simulink model "EKF_SIL_02_newdelIpsOOSM"  (R2014a)
settings: Solver=ode45  StartTime=0.0  StopTime=50  RelTol=1e-3
model workspace: external: MATLAB File InitOOSM.m (data not in the file)
undefined symbols (not defined in the file): Cov_nu, Cov_r, e_force_x, e_force_y, e_force_z, ieps, ita, n, P_0, P_k, p_x, p_y, p_z, parameter_gravitation, rho, rho_c, sig_f, sig_tau, t_delta, t_Kalman, t_RobotSense, tau_1, tau_2, tau_3, U_n_d, X_a_0, x_k
libraries: simulink x9, dspmtrx3 x4, aerolibtransform2 x2, visionsinks x1
(part 3 of 6)

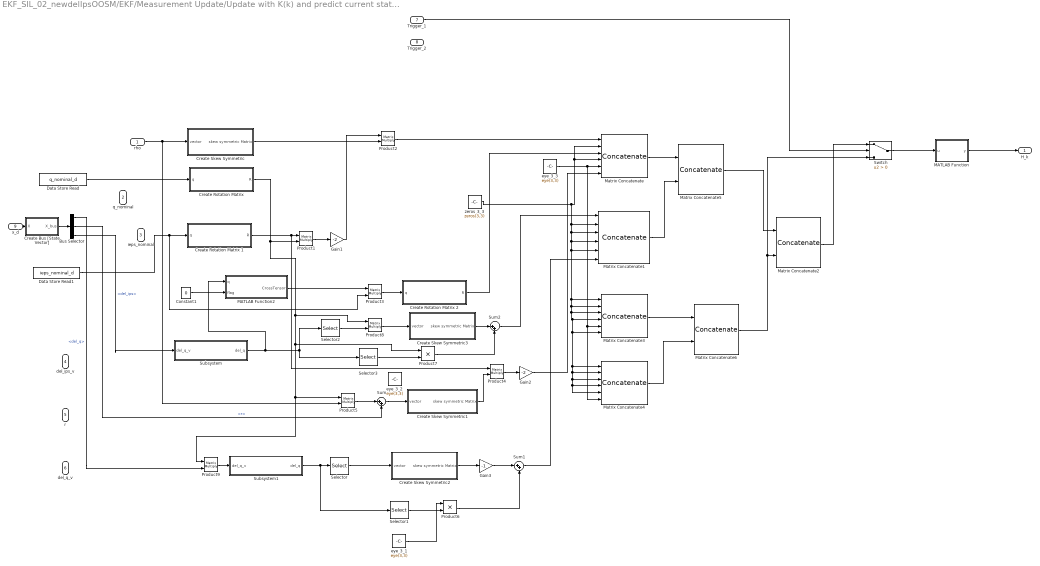
== system EKF_SIL_02_newdelIpsOOSM/EKF/Measurement Update/Update with K(k) and predict current state/Create H_k ==
  rho : Inport
  q_nominal : Inport  Port=2
  ieps_nominal : Inport  Port=3
  del_ips_v : Inport  Port=4
  r : Inport  Port=5
  del_q_v : Inport  Port=6
  Trigger_1 : Inport  Port=7
  Trigger_2 : Inport  Port=8
  x_d : Inport  Port=9
  Bus Selector : BusSelector  OutputSignals=del_q,r,del_ips
  Constant1 : Constant  Value=0
  Create Bus [State Vector] : Subsystem
  "Create Rotation Matrix " : Subsystem
  Create Rotation Matrix 1 : Subsystem
  Create Rotation Matrix 2 : Subsystem
  Create Skew Symmetric : Subsystem
  Create Skew Symmetric1 : Subsystem
  Create Skew Symmetric2 : Subsystem
  Create Skew Symmetric3 : Subsystem
  Data Store Read : DataStoreRead  DataStoreName=q_nominal_d
  Data Store Read1 : DataStoreRead  DataStoreName=ieps_nominal_d
  Gain1 : Gain  Gain=-2
  Gain2 : Gain  Gain=-2
  Gain3 : Gain  Gain=-1
  MATLAB Function : MATLAB Function  TreatAsAtomicUnit=on
      settings: PermitHierarchicalResolution=ParametersOnly
  MATLAB Function2 : MATLAB Function  TreatAsAtomicUnit=on
      settings: PermitHierarchicalResolution=ParametersOnly
  Matrix Concatenate{,1,3..4} (4 alike) : Concatenate  NumInputs=6  Mode=Multidimensional array  ConcatenateDimension=2
  Matrix Concatenate2 : Concatenate  Mode=Multidimensional array
  Matrix Concatenate5 : Concatenate  Mode=Multidimensional array
  Matrix Concatenate6 : Concatenate  Mode=Multidimensional array
  Product{1..5,8..9} (7 alike) : Product  Multiplication=Matrix(*)
  Product6 : Product
  Product7 : Product
  Selector : Selector  InputPortWidth=4  Indices=[1:3]
  Selector1 : Selector  InputPortWidth=4  Indices=4
  Selector2 : Selector  InputPortWidth=4  Indices=[1:3]
  Selector3 : Selector  InputPortWidth=4  Indices=4
  Subsystem : Subsystem
  Subsystem1 : Subsystem
  Sum : Sum  Inputs=|++
  Sum1 : Sum  Inputs=|++
  Sum2 : Sum  Inputs=|++
  Switch : Switch  Criteria=u2 > Threshold  AllowDiffInputSizes=on
  eye_3_1 : Constant  Value=eye(3,3)
  eye_3_2 : Constant  Value=eye(3,3)
  eye_3_3 : Constant  Value=eye(3,3)
  zeros_3_3 : Constant  Value=zeros(3,3)
  H_k : Outport
  wires:
  Data Store Read/1 -> "Create Rotation Matrix "/1(q)
  Switch/1 -> MATLAB Function/1(u)
  eye_3_3/1 -> Matrix Concatenate4/6, Matrix Concatenate3/5, Matrix Concatenate/5
  Create Skew Symmetric/1(skew symmetric Matrix) -> Product2/2
  rho/1 -> Product5/2, Create Skew Symmetric/1(vector)
  Create Rotation Matrix 1/1(R) -> Product4/1, Product1/1
  Product1/1 -> Gain1/1
  Gain1/1 -> Product2/1
  Product2/1 -> Matrix Concatenate/1
  Bus Selector/3 -> Subsystem/1(del_q_v)  "<del_ips>"
  Constant1/1 -> MATLAB Function2/2(flag)
  MATLAB Function2/1(CrossTensor) -> Product3/1
  Data Store Read1/1 -> Product3/2, Create Rotation Matrix 1/1(q)
  Create Rotation Matrix 2/1(R) -> Matrix Concatenate/3
  "Create Rotation Matrix "/1(R) -> Product7/1, Product9/1, Product5/1, Product8/1, Product1/2
  Product5/1 -> Sum/1
  Bus Selector/2 -> Sum/2  "<r>"
  Gain2/1 -> Matrix Concatenate/6
  Subsystem1/1(del_q) -> Selector1/1, Selector/1
  Selector/1 -> Create Skew Symmetric2/1(vector)
  Create Skew Symmetric2/1(skew symmetric Matrix) -> Gain3/1
  Selector1/1 -> Product6/2
  eye_3_1/1 -> Product6/1
  Gain3/1 -> Sum1/1
  Product6/1 -> Sum1/2
  Sum1/1 -> Matrix Concatenate1/6
  Selector2/1 -> Product8/2
  Create Skew Symmetric3/1(skew symmetric Matrix) -> Sum2/1
  Selector3/1 -> Product7/2
  Product7/1 -> Sum2/2
  Sum2/1 -> Matrix Concatenate1/1
  Sum/1 -> Create Skew Symmetric1/1(vector)
  Create Skew Symmetric1/1(skew symmetric Matrix) -> Product4/2
  Product3/1 -> Create Rotation Matrix 2/1(q)
  zeros_3_3/1 -> Matrix Concatenate3/6, Matrix Concatenate4/1, Matrix Concatenate4/5, Matrix Concatenate4/4, Matrix Concatenate4/3, Matrix Concatenate4/2, Matrix Concatenate3/4, Matrix Concatenate3/3, Matrix Concatenate3/2, Matrix Concatenate3/1, Matrix Concatenate1/5, Matrix Concatenate1/4, Matrix Concatenate1/3, Matrix Concatenate1/2, Matrix Concatenate/4, Matrix Concatenate/2
  Matrix Concatenate1/1 -> Matrix Concatenate5/2
  Matrix Concatenate4/1 -> Matrix Concatenate6/2
  Subsystem/1(del_q) -> MATLAB Function2/1(q), Selector2/1, Selector3/1
  Bus Selector/1 -> Product9/2  "<del_q>"
  Product9/1 -> Subsystem1/1(del_q_v)
  Product8/1 -> Create Skew Symmetric3/1(vector)
  Product4/1 -> Gain2/1
  Matrix Concatenate/1 -> Matrix Concatenate5/1
  Matrix Concatenate3/1 -> Matrix Concatenate6/1
  Trigger_1/1 -> Switch/2
  Matrix Concatenate5/1 -> Matrix Concatenate2/1
  Matrix Concatenate6/1 -> Switch/3, Matrix Concatenate2/2
  Matrix Concatenate2/1 -> Switch/1
  MATLAB Function/1(y) -> H_k/1
  Create Bus [State Vector]/1(X_bus) -> Bus Selector/1
  x_d/1 -> Create Bus [State Vector]/1(X)

== system EKF_SIL_02_newdelIpsOOSM/EKF/Measurement Update/Update with K(k) and predict current state/Create S_k ==
  ita_nominal : Inport
  trig_1 : Inport  Port=2
  trig_2 : Inport  Port=3
  q_nominal : Inport  Port=4
  cov_r : Inport  Port=5
  cov_nu : Inport  Port=6
  Constant : Constant  Value=1e-4*eye(6,6)
  Constant1 : Constant  Value=zeros(6,6)
  Data Store Read : DataStoreRead  DataStoreName=q_nominal_d
  Matrix Concatenate1 : Concatenate  Mode=Multidimensional array
  Matrix Concatenate5 : Concatenate  Mode=Multidimensional array  ConcatenateDimension=2
  Matrix Concatenate6 : Concatenate  Mode=Multidimensional array  ConcatenateDimension=2
  Measurement noise covariance : MATLAB Function  TreatAsAtomicUnit=on
      settings: PermitHierarchicalResolution=ParametersOnly
  Switch : Switch  Criteria=u2 > Threshold  AllowDiffInputSizes=on
  S_k : Outport
  wires:
  ita_nominal/1 -> Measurement noise covariance/2(ita_nominal)
  cov_nu/1 -> Measurement noise covariance/4(cov_nu)
  cov_r/1 -> Measurement noise covariance/3(cov_r)
  Measurement noise covariance/1(S) -> Matrix Concatenate5/1, Switch/3
  trig_1/1 -> Switch/2
  Constant1/1 -> Matrix Concatenate6/1, Matrix Concatenate5/2
  Constant/1 -> Matrix Concatenate6/2
  Switch/1 -> S_k/1
  Matrix Concatenate1/1 -> Switch/1
  Matrix Concatenate5/1 -> Matrix Concatenate1/1
  Matrix Concatenate6/1 -> Matrix Concatenate1/2
  Data Store Read/1 -> Measurement noise covariance/1(q_nominal)

== system EKF_SIL_02_newdelIpsOOSM/EKF/Measurement Update/Update with K(k) and predict current state/Create X_a from X ==
  q_nominal : Inport
  X : Inport  Port=2
  ieps_nominal : Inport  Port=3
  Bus Creator1 : BusCreator
  Bus Creator2 : BusCreator  Inputs=6
  Bus Creator3 : BusCreator
  Bus Selector2 : BusSelector  OutputSignals=del_q,del_ips
  Bus Selector3 : BusSelector  OutputSignals=omega,r,r_dot,rho_c
  Create Bus [State Vector] : Subsystem
  "Create q_nominal " : Subsystem
  Create q_nominal 1 : Subsystem
  Demux : Demux
  Demux1 : Demux
  Display2 : Display
  Signal Conversion : SignalConversion
  X_a(k+1) : Outport
  X_a(internal) : Outport  Port=2
  "X(reduced) " : Outport  Port=3
  wires:
  Bus Selector3/3 -> Bus Creator2/4  "<r_dot>"
  Demux/1 -> Bus Creator3/1  "q_est_1"
  Bus Selector3/2 -> Bus Creator2/3  "<r>"
  Bus Creator3/1 -> Bus Creator2/1  "q_est"
  Create Bus [State Vector]/1(X_bus) -> "X(reduced) "/1, Bus Selector3/1, Bus Selector2/1
  X/1 -> Create Bus [State Vector]/1(X)
  Bus Selector3/1 -> Bus Creator2/2  "<omega>"
  Demux/2 -> Bus Creator3/2  "q_est_2"
  Demux/4 -> Bus Creator3/4  "q_est_0"
  Demux/3 -> Bus Creator3/3  "q_est_3"
  Bus Selector2/1 -> "Create q_nominal "/1(del_q)  "<del_q>"
  q_nominal/1 -> "Create q_nominal "/2(q_nominal)
  "Create q_nominal "/1(q_est) -> Demux/1
  Bus Creator2/1 -> Signal Conversion/1, X_a(internal)/1
  Bus Selector2/2 -> Create q_nominal 1/1(del_q)  "<del_ips>"
  ieps_nominal/1 -> Create q_nominal 1/2(q_nominal)
  Bus Selector3/4 -> Bus Creator2/5  "<rho_c>"
  Demux1/1 -> Bus Creator1/1  "ieps_est_1"
  Bus Creator1/1 -> Bus Creator2/6  "ieps_est"
  Demux1/2 -> Bus Creator1/2  "ieps_est_2"
  Demux1/4 -> Bus Creator1/4  "ieps_est_0"
  Demux1/3 -> Bus Creator1/3  "ieps_est_3"
  Create q_nominal 1/1(q_est) -> Display2/1, Demux1/1
  Signal Conversion/1 -> X_a(k+1)/1

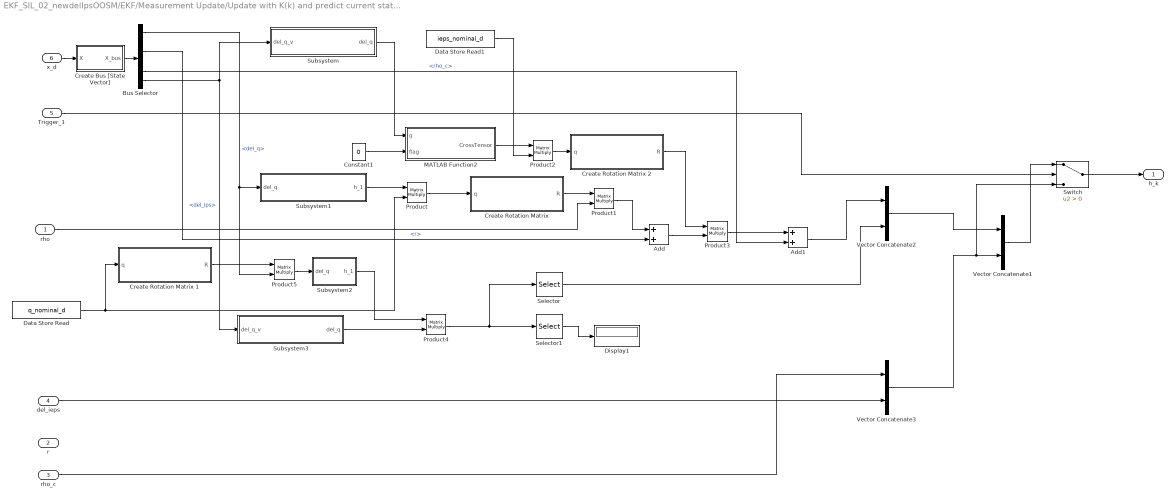
== system EKF_SIL_02_newdelIpsOOSM/EKF/Measurement Update/Update with K(k) and predict current state/Create h ==
  rho : Inport
  r : Inport  Port=2
  rho_c : Inport  Port=3
  "del_ieps " : Inport  Port=4
  Trigger_1 : Inport  Port=5
  x_d : Inport  Port=6
  Add : Sum
  Add1 : Sum
  Bus Selector : BusSelector  OutputSignals=del_q,omega,r,r_dot,rho_c,del_ips
  Constant1 : Constant  Value=0
  Create Bus [State Vector] : Subsystem
  "Create Rotation Matrix " : Subsystem
  Create Rotation Matrix 1 : Subsystem
  Create Rotation Matrix 2 : Subsystem
  Data Store Read : DataStoreRead  DataStoreName=q_nominal_d
  Data Store Read1 : DataStoreRead  DataStoreName=ieps_nominal_d
  Display1 : Display
  MATLAB Function2 : MATLAB Function  TreatAsAtomicUnit=on
      settings: PermitHierarchicalResolution=ParametersOnly
  Product{,1..5} (6 alike) : Product  Multiplication=Matrix(*)
  Selector : Selector  InputPortWidth=4  Indices=[1:3]
  Selector1 : Selector  InputPortWidth=4  Indices=4
  Subsystem : Subsystem
  Subsystem1 : Subsystem
  Subsystem2 : Subsystem
  Subsystem3 : Subsystem
  Switch : Switch  Criteria=u2 > Threshold  AllowDiffInputSizes=on
  Vector Concatenate1 : Concatenate
  Vector Concatenate2 : Concatenate
  Vector Concatenate3 : Concatenate
  h_k : Outport
  wires:
  rho/1 -> Product1/2
  Data Store Read/1 -> Product/2, Create Rotation Matrix 1/1(q)
  "Create Rotation Matrix "/1(R) -> Product1/1
  Product/1 -> "Create Rotation Matrix "/1(q)
  Subsystem1/1(h_1) -> Product/1
  Product1/1 -> Add/1
  rho_c/1 -> Vector Concatenate3/1
  "del_ieps "/1 -> Vector Concatenate3/2
  Create Rotation Matrix 2/1(R) -> Product3/1
  Product3/1 -> Add1/1
  Add/1 -> Product3/2
  Add1/1 -> Vector Concatenate2/1
  Product4/1 -> Selector1/1, Selector/1
  Selector1/1 -> Display1/1
  Create Rotation Matrix 1/1(R) -> Product5/1
  Product5/1 -> Subsystem2/1(del_q)
  Subsystem2/1(h_1) -> Product4/1
  Selector/1 -> Vector Concatenate2/2
  Trigger_1/1 -> Switch/2
  Vector Concatenate2/1 -> Vector Concatenate1/1
  Vector Concatenate3/1 -> Switch/3, Vector Concatenate1/2
  Switch/1 -> h_k/1
  Vector Concatenate1/1 -> Switch/1
  x_d/1 -> Create Bus [State Vector]/1(X)
  Bus Selector/1 -> Product5/2, Subsystem1/1(del_q)  "<del_q>"
  Bus Selector/3 -> Add/2  "<r>"
  Bus Selector/5 -> Add1/2  "<rho_c>"
  Bus Selector/6 -> Subsystem3/1(del_q_v), Subsystem/1(del_q_v)  "<del_ips>"
  Subsystem3/1(del_q) -> Product4/2
  Create Bus [State Vector]/1(X_bus) -> Bus Selector/1
  Constant1/1 -> MATLAB Function2/2(flag)
  Subsystem/1(del_q) -> MATLAB Function2/1(q)
  MATLAB Function2/1(CrossTensor) -> Product2/1
  Product2/1 -> Create Rotation Matrix 2/1(q)
  Data Store Read1/1 -> Product2/2

== matlab function EKF_SIL_02_newdelIpsOOSM/EKF/OOSM_KF/OOSM_KF/State Propagation/MATLAB Function ==
  data: X_a input; Phi output; n input; t_Kalman input; p input; M input; V input; om_EE input
%Function: fn_Create_Phi()
%Inputs: X_a - 23-state vector,
%        n - angular velocity of spacecrafts,
%        t_delta - sampling time
%Outputs: [Phi] (State-propagation Matrix)
%Functionality: Generates the State Propagation matrix
%Author: Hrishik Mishra
function Phi  = fn_Create_Phi(X_a,n,t_Kalman,p,M,V,om_EE)
    Phi_t = fn_Create_Phi_t(n,t_Kalman);
    Phi_r = fn_Create_Phi_r(X_a,p, t_Kalman);    
    Phi_rho_c = expm(fn_VectorToSkewSymmetricTensor(V(4:6))*t_Kalman);
    Phi_ieps = expm(-fn_VectorToSkewSymmetricTensor(om_EE*t_Kalman));
    Phi_robot = [Phi_rho_c,zeros(3,3);zeros(3,3),Phi_ieps];
    
    Phi = [Phi_r, zeros(6,12);zeros(6,6),Phi_t,zeros(6,6);zeros(6,12),Phi_robot];

end
%Create state propagation matrix of the whole system

%Function: fn_Create_Phi_r()
%Inputs: X_a - 23-state vector,
%Outputs: [Phi_r] (State-propagation Matrix for Rotation component)
%Functionality: Generates the State Propagation matrix for Rotation
%component
%Author: Hrishik Mishra
function [Phi_r] = fn_Create_Phi_r(X_a,p,t_Kalman) 
    Phi_r = zeros(6,6);
    omega = X_a(5:7);
    M = fn_Create_M(p,omega);   
    
    A = [-fn_VectorToSkewSymmetricTensor(omega),0.5*eye(3,3);zeros(3,3),M];
    Phi_r = expm(A*t_Kalman);
%     phi_r11 = fn_Create_phi_r11(omega,t_delta);
%     phi_r12 = fn_Create_phi_r12(omega,M,t_delta);
%     phi_r22 = fn_Create_phi_r22(omega,t_delta,M);
%     phi_r13 = fn_Create_phi_r13(omega,t_delta,M,N);
%     phi_r23 = fn_Create_phi_r23(omega,t_delta,M,N);
%     Phi_r = [phi_r11, phi_r12, phi_r13;zeros(3,3),phi_r22,phi_r23;zeros(3,3),zeros(3,3),eye(3,3)];
%     

end
%Function: fn_Create_M()
%Inputs: p - Inertial ratios 
%        omega - angular velocity between Chaser Grasping frame and Chaser
%        CoM
%Outputs: M (Linearized model matrix for inertial parameters)
%Functionality: Generates M
%Author: Hrishik Mishra
function M = fn_Create_M(p,omega)
    %#Codegen
    
    M = [0, p(1)*omega(3), p(1)*omega(2); p(2)*omega(3), 0, p(2)*omega(1); p(3)*omega(2),p(3)*omega(1),0];
end
%Function: fn_Create_N()
%Inputs: omega - angular velocity between Chaser Grasping frame and Chaser
%        CoM
%Outputs: N (Linearized model matrix for inertial parameters)
%Functionality: Generates M
%Author: Hrishik Mishra
function N = fn_Create_N(omega)
%
    N = [omega(2)*omega(3), 0, 0; 0, omega(1)*omega(3), 0; 0, 0, omega(1)*omega(2)];
end

%%
%Function: fn_Create_Phi_t()
%Inputs: n - angular velocity of Chaser/Target (almost same)
%        t_delta - sampling time
%Outputs: Phi_t (State Transition Matrix for Translation component)
%Functionality: Generates Phi_t
%Author: Hrishik Mishra
function Phi_t = fn_Create_Phi_t(n,t_delta)
%
    Phi_t12 = [t_delta, n*t_delta^2,0;0, t_delta, 0;0,0,t_delta];
    Phi_t22 = eye(3,3) - 2*fn_VectorToSkewSymmetricTensor([0;0;n])*t_delta;
    
    Phi_t = [eye(3,3),Phi_t12;zeros(3,3),Phi_t22];
    
end

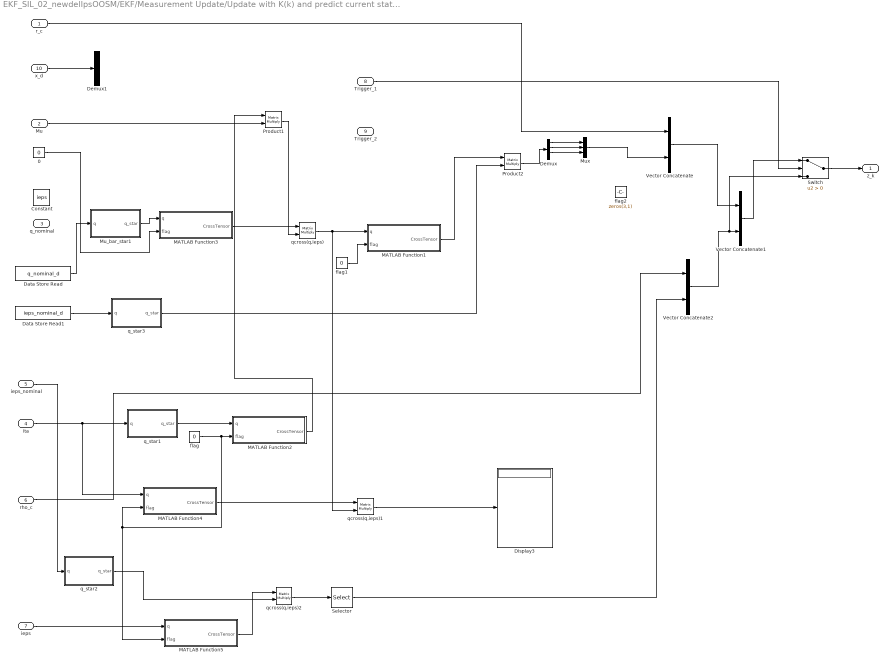
== system EKF_SIL_02_newdelIpsOOSM/EKF/Measurement Update/Update with K(k) and predict current state/Create observation ==
  r_c : Inport
  Mu : Inport  Port=2
  q_nominal : Inport  Port=3
  ita : Inport  Port=4
  ieps_nominal : Inport  Port=5
  rho_c : Inport  Port=6
  ieps : Inport  Port=7
  Trigger_1 : Inport  Port=8
  Trigger_2 : Inport  Port=9
  x_d : Inport  Port=10
  0 : Constant  Value=0
  Constant : Constant  Value=ieps
  Data Store Read : DataStoreRead  DataStoreName=q_nominal_d
  Data Store Read1 : DataStoreRead  DataStoreName=ieps_nominal_d
  Demux : Demux
  Demux1 : Demux  Outputs=6
  Display3 : Display
  MATLAB Function1 : MATLAB Function  TreatAsAtomicUnit=on
      settings: PermitHierarchicalResolution=ParametersOnly
  MATLAB Function2 : MATLAB Function  TreatAsAtomicUnit=on
      settings: PermitHierarchicalResolution=ParametersOnly
  MATLAB Function3 : MATLAB Function  TreatAsAtomicUnit=on
      settings: PermitHierarchicalResolution=ParametersOnly
  MATLAB Function4 : MATLAB Function  TreatAsAtomicUnit=on
      settings: PermitHierarchicalResolution=ParametersOnly
  MATLAB Function5 : MATLAB Function  TreatAsAtomicUnit=on
      settings: PermitHierarchicalResolution=ParametersOnly
  Mu_bar_star1 : Subsystem
  Mux : Mux  Inputs=3
  Product1 : Product  Multiplication=Matrix(*)
  Product2 : Product  Multiplication=Matrix(*)
  Selector : Selector  InputPortWidth=4  Indices=[1:3]
  Switch : Switch  Criteria=u2 > Threshold  AllowDiffInputSizes=on
  Vector Concatenate : Concatenate
  Vector Concatenate1 : Concatenate
  Vector Concatenate2 : Concatenate
  flag : Constant  Value=0
  flag1 : Constant  Value=0
  flag2 : Constant  Value=zeros(3,1)
  q_star1 : Subsystem
  q_star2 : Subsystem
  q_star3 : Subsystem
  qcross(q,ieps) : Product  Multiplication=Matrix(*)
  qcross(q,ieps)1 : Product  Multiplication=Matrix(*)
  qcross(q,ieps)2 : Product  Multiplication=Matrix(*)
  z_k : Outport
  wires:
  MATLAB Function2/1(CrossTensor) -> Product1/1
  flag/1 -> MATLAB Function2/2(flag), MATLAB Function4/2(flag), MATLAB Function5/2(flag)
  q_star1/1(q_star) -> MATLAB Function2/1(q)
  ita/1 -> MATLAB Function4/1(q), q_star1/1(q)
  Demux/1 -> Mux/1
  Demux/2 -> Mux/2
  Demux/3 -> Mux/3
  Mux/1 -> Vector Concatenate/2
  0/1 -> MATLAB Function3/2(flag)
  r_c/1 -> Vector Concatenate/1
  MATLAB Function1/1(CrossTensor) -> Product2/1
  Product2/1 -> Demux/1
  MATLAB Function3/1(CrossTensor) -> qcross(q,ieps)/1
  ieps_nominal/1 -> q_star2/1(q)
  qcross(q,ieps)/1 -> qcross(q,ieps)1/2, MATLAB Function1/1(q)
  Mu/1 -> Product1/2
  MATLAB Function4/1(CrossTensor) -> qcross(q,ieps)1/1
  qcross(q,ieps)1/1 -> Display3/1
  flag1/1 -> MATLAB Function1/2(flag)
  rho_c/1 -> Vector Concatenate2/1
  q_star2/1(q_star) -> qcross(q,ieps)2/2
  MATLAB Function5/1(CrossTensor) -> qcross(q,ieps)2/1
  ieps/1 -> MATLAB Function5/1(q)
  qcross(q,ieps)2/1 -> Selector/1
  Selector/1 -> Vector Concatenate2/2
  Mu_bar_star1/1(q_star) -> MATLAB Function3/1(q)
  Product1/1 -> qcross(q,ieps)/2
  Vector Concatenate/1 -> Vector Concatenate1/1
  Trigger_1/1 -> Switch/2
  Vector Concatenate2/1 -> Switch/3, Vector Concatenate1/2
  Switch/1 -> z_k/1
  Vector Concatenate1/1 -> Switch/1
  x_d/1 -> Demux1/1
  Data Store Read/1 -> Mu_bar_star1/1(q)
  q_star3/1(q_star) -> Product2/2
  Data Store Read1/1 -> q_star3/1(q)

== system EKF_SIL_02_newdelIpsOOSM/EKF/Measurement Update/Update with K(k) and predict current state/K*H ==
  H : Inport
  K : Inport  Port=2
  Sd : Inport  Port=3
  MATLAB Function : MATLAB Function  TreatAsAtomicUnit=on
      settings: PermitHierarchicalResolution=ParametersOnly
  K*Sd*K' : Outport
  wires:
  K/1 -> MATLAB Function/1(K)
  MATLAB Function/1(y) -> K*Sd*K'/1
  Sd/1 -> MATLAB Function/2(Sd)

== system EKF_SIL_02_newdelIpsOOSM/EKF/Measurement Update/Update with K(k) and predict current state/Kalman gain ==
  H_k : Inport
  P_pre : Inport  Port=2
  S_k : Inport  Port=3
  P_d : Inport  Port=4
  U : Inport  Port=5
  UF : Inport  Port=6
  trig_1 : Inport  Port=7
  Display3 : Display
  MATLAB Function : MATLAB Function  TreatAsAtomicUnit=on
      settings: PermitHierarchicalResolution=ParametersOnly
  Math Function1 : Math  Operator=log10  SaturateOnIntegerOverflow=on
  Scope : Scope
      settings: YMin=-1.61  YMax=-1.41  SaveName=ScopeData22
  Selector : Selector  NumberOfDimensions=2  InputPortWidth=3  IndexOptions=Index vector (dialog),Index vector (dialog)  Indices=[1:6],[1:6]  OutputSizes=1,1
  Sum of Elements : Sum  Inputs=+
  K : Outport
  H.P(k|k-1).H' + S_k : Outport  Port=2
  wires:
  H_k/1 -> MATLAB Function/1(H)
  P_pre/1 -> MATLAB Function/2(P_pre)
  Selector/1 -> Sum of Elements/1
  Sum of Elements/1 -> Math Function1/1
  Math Function1/1 -> Scope/1
  S_k/1 -> MATLAB Function/3(S_k)
  MATLAB Function/1(K) -> K/1
  MATLAB Function/2(Cov_x_y) -> Selector/1, H.P(k|k-1).H' + S_k/1
  P_d/1 -> MATLAB Function/5(P_d)
  U/1 -> MATLAB Function/7(U)
  UF/1 -> MATLAB Function/4(UF)
  trig_1/1 -> MATLAB Function/6(trig_1)

== system EKF_SIL_02_newdelIpsOOSM/EKF/Measurement Update/Update with K(k) and predict current state/MhDist ==
  x : Inport
  Var : Inport  Port=2
  MATLAB Function : MATLAB Function  TreatAsAtomicUnit=on
      settings: PermitHierarchicalResolution=ParametersOnly
  d^2 : Outport
  wires:
  MATLAB Function/1(y) -> d^2/1
  x/1 -> MATLAB Function/1(x)
  Var/1 -> MATLAB Function/2(Var)

== system EKF_SIL_02_newdelIpsOOSM/EKF/Measurement Update/Update with K(k) and predict current state/Outlier rejector ==
  Computed K : Inport
  X^2 : Inport  Port=2
  Chi_threshold : Constant  Value=1000
  Relational Operator : RelationalOperator  Operator=<  OutDataTypeStr=boolean
  Scope : Scope
      settings: ShowLegends=on  SaveName=ScopeData31
  Switch : Switch  Criteria=u2 > Threshold
  zeros(12,) : Constant  Value=zeros(12,6)
  K (outlier_checked) : Outport
  wires:
  Computed K/1 -> Switch/1
  X^2/1 -> Relational Operator/1
  Chi_threshold/1 -> Relational Operator/2
  Relational Operator/1 -> Switch/2, Scope/1  "Outlier rejector (Not)"
  Switch/1 -> K (outlier_checked)/1
  zeros(12,)/1 -> Switch/3

== system EKF_SIL_02_newdelIpsOOSM/EKF/Measurement Update/Update with K(k) and predict current state/Subsystem ==
  residual : Inport
  K : Inport  Port=2
  MATLAB Function : MATLAB Function  TreatAsAtomicUnit=on
      settings: PermitHierarchicalResolution=ParametersOnly
  K(z-h(x)) : Outport
  wires:
  MATLAB Function/1(y) -> K(z-h(x))/1
  K/1 -> MATLAB Function/1(K)
  residual/1 -> MATLAB Function/2(del_x)

== system EKF_SIL_02_newdelIpsOOSM/EKF/Measurement Update/Update with K(k) and predict current state/Subsystem1 ==
  residual : Inport
  HPH+R : Inport  Port=2
  UF : Inport  Port=3
  Pd : Inport  Port=4
  U : Inport  Port=5
  H : Inport  Port=6
  x_d : Inport  Port=7
  K : Inport  Port=8
  Phi : Inport  Port=9
  Enable : EnablePort
  MATLAB Function : MATLAB Function  TreatAsAtomicUnit=on
      settings: PermitHierarchicalResolution=ParametersOnly
  U_k+1 : Outport
  x_d_n+1 : Outport  Port=2
  P_d_n_1 : Outport  Port=3
  wires:
  residual/1 -> MATLAB Function/2(del_x)
  HPH+R/1 -> MATLAB Function/1(Sk)
  MATLAB Function/1(U1) -> U_k+1/1
  UF/1 -> MATLAB Function/3(UF)
  Pd/1 -> MATLAB Function/4(Pd)
  U/1 -> MATLAB Function/5(U)
  H/1 -> MATLAB Function/6(H)
  x_d/1 -> MATLAB Function/7(x_d)
  K/1 -> MATLAB Function/8(K)
  Phi/1 -> MATLAB Function/9(Phi)
  MATLAB Function/2(xd) -> x_d_n+1/1
  MATLAB Function/3(Pd1) -> P_d_n_1/1

== system EKF_SIL_02_newdelIpsOOSM/EKF/OOSM_KF/OOSM_KF/Create Bus [State Vector,X_a] ==
  X : Inport
  Bus Creator{1,3..5} (4 alike) : BusCreator  Inputs=3
  Bus Creator2 : BusCreator
  Bus Creator6 : BusCreator  Inputs=6
  Bus Creator7 : BusCreator
  Demux1 : Demux  Outputs=20
  X_bus : Outport
  wires:
  Bus Creator2/1 -> Bus Creator6/1  "q_est"
  Bus Creator3/1 -> Bus Creator6/2  "omega"
  Bus Creator4/1 -> Bus Creator6/3  "r"
  Bus Creator5/1 -> Bus Creator6/4  "r_dot"
  Bus Creator6/1 -> X_bus/1
  X/1 -> Demux1/1
  Demux1/1 -> Bus Creator2/1  "q_est_1"
  Demux1/2 -> Bus Creator2/2  "q_est_2"
  Demux1/3 -> Bus Creator2/3  "q_est_3"
  Demux1/4 -> Bus Creator2/4  "q_est_0"
  Demux1/5 -> Bus Creator3/1  "omega_x"
  Demux1/6 -> Bus Creator3/2  "omega_y"
  Demux1/7 -> Bus Creator3/3  "omega_z"
  Demux1/8 -> Bus Creator4/1  "r_x"
  Demux1/9 -> Bus Creator4/2  "r_y"
  Demux1/10 -> Bus Creator4/3  "r_z"
  Demux1/11 -> Bus Creator5/1  "r_x_dot"
  Demux1/12 -> Bus Creator5/2  "r_y_dot"
  Demux1/13 -> Bus Creator5/3  "r_z_dot"
  Demux1/14 -> Bus Creator1/1  "rho_c_x"
  Demux1/15 -> Bus Creator1/2  "rho_c_y"
  Demux1/16 -> Bus Creator1/3  "rho_c_z"
  Demux1/17 -> Bus Creator7/1  "ieps_1"
  Demux1/18 -> Bus Creator7/2  "ieps_2"
  Demux1/19 -> Bus Creator7/3  "ieps_3"
  Demux1/20 -> Bus Creator7/4  "ieps_0"
  Bus Creator1/1 -> Bus Creator6/5  "rho_c"
  Bus Creator7/1 -> Bus Creator6/6  "ieps"

== system EKF_SIL_02_newdelIpsOOSM/EKF/OOSM_KF/OOSM_KF/Create Bus [State Vector] ==
  X : Inport
  Bus Creator{1..5,7} (6 alike) : BusCreator  Inputs=3
  Bus Creator6 : BusCreator  Inputs=6
  Demux1 : Demux  Outputs=18
  X_bus : Outport
  wires:
  Demux1/4 -> Bus Creator3/1  "omega_x"
  Bus Creator2/1 -> Bus Creator6/1  "del_q"
  Demux1/8 -> Bus Creator4/2  "r_y"
  Demux1/6 -> Bus Creator3/3  "omega_z"
  Demux1/7 -> Bus Creator4/1  "r_x"
  Demux1/10 -> Bus Creator5/1  "r_x_dot"
  Bus Creator3/1 -> Bus Creator6/2  "omega"
  Demux1/3 -> Bus Creator2/3  "del_q_3"
  Demux1/1 -> Bus Creator2/1  "del_q_1"
  Demux1/11 -> Bus Creator5/2  "r_y_dot"
  Demux1/12 -> Bus Creator5/3  "r_z_dot"
  Demux1/2 -> Bus Creator2/2  "del_q_2"
  Demux1/5 -> Bus Creator3/2  "omega_y"
  Demux1/9 -> Bus Creator4/3  "r_z"
  Bus Creator4/1 -> Bus Creator6/3  "r"
  Bus Creator5/1 -> Bus Creator6/4  "r_dot"
  Bus Creator6/1 -> X_bus/1
  X/1 -> Demux1/1
  Demux1/13 -> Bus Creator1/1  "rho_c_x"
  Demux1/14 -> Bus Creator1/2  "rho_c_y"
  Demux1/15 -> Bus Creator1/3  "rho_c_z"
  Demux1/16 -> Bus Creator7/1  "del_ieps_1"
  Demux1/17 -> Bus Creator7/2
  Demux1/18 -> Bus Creator7/3  "del_ips_3"
  Bus Creator1/1 -> Bus Creator6/5  "rho_c"
  Bus Creator7/1 -> Bus Creator6/6  "del_ips"

== system EKF_SIL_02_newdelIpsOOSM/EKF/OOSM_KF/OOSM_KF/Create X from X_a1 ==
  X_a(k) : Inport
  q_nominal(k) : Inport  Port=2
  ieps_nominal : Inport  Port=3
  Bus Creator1 : BusCreator  Inputs=6
  Bus Selector3 : BusSelector  OutputSignals=q_est,omega,r,r_dot,rho_c,ieps
  Bus Selector5 : BusSelector  OutputSignals=q_est,ieps
  Create Bus [State Vector,X_a] : Subsystem
  Create Bus [State Vector] : Subsystem
  Create del_q [body] : Subsystem
  Create del_q [inertial] : Subsystem
  IC : InitialCondition  Value=[X_a_0]
  X(k) : Outport
  q(k) : Outport  Port=2
  ieps(k) : Outport  Port=3
  wires:
  Create Bus [State Vector,X_a]/1(X_bus) -> Bus Selector3/1, Bus Selector5/1
  Create del_q [body]/1(del_q) -> Bus Creator1/1  "del_q"
  Bus Selector3/2 -> Bus Creator1/2  "<omega>"
  Bus Selector3/3 -> Bus Creator1/3  "<r>"
  Bus Selector3/4 -> Bus Creator1/4  "<r_dot>"
  Bus Creator1/1 -> Create Bus [State Vector]/1(X)
  Bus Selector5/1 -> Create del_q [body]/1(q)  "<q_est>"
  Create Bus [State Vector]/1(X_bus) -> X(k)/1
  X_a(k)/1 -> IC/1
  IC/1 -> Create Bus [State Vector,X_a]/1(X)
  Bus Selector3/1 -> q(k)/1  "<q_est>"
  q_nominal(k)/1 -> Create del_q [body]/2(q_nominal)
  ieps_nominal/1 -> Create del_q [inertial]/2(q_nominal)
  Bus Selector5/2 -> Create del_q [inertial]/1(q)  "<ieps>"
  Bus Selector3/5 -> Bus Creator1/5  "<rho_c>"
  Create del_q [inertial]/1(del_q) -> Bus Creator1/6  "del_ieps"
  Bus Selector3/6 -> ieps(k)/1  "<ieps>"

== system EKF_SIL_02_newdelIpsOOSM/EKF/OOSM_KF/OOSM_KF/State Propagation ==
  "X_a(t)\t" : Inport
  V : Inport  Port=2
  Bus Selector : BusSelector  OutputSignals=ieps
  Create M : Subsystem
  Create Rotation Matrix 1 : Subsystem
  MATLAB Function : MATLAB Function  TreatAsAtomicUnit=on
      settings: PermitHierarchicalResolution=ParametersOnly
  Math Function : Math  Operator=transpose  SaturateOnIntegerOverflow=on
  Product : Product  Multiplication=Matrix(*)
  Selector : Selector  InputPortWidth=6  Indices=[4:6]
  Signal Specification : SignalSpecification  Dimensions=[18,18]
  n : Constant  Value=n
  p : Constant  Value=[p_x;p_y;p_z]
  "t_Kalman " : Constant  Value=t_Kalman
  Phi : Outport
  wires:
  p/1 -> Create M/2(p), MATLAB Function/4(p)
  n/1 -> MATLAB Function/2(n)
  "t_Kalman "/1 -> MATLAB Function/3(t_Kalman)
  MATLAB Function/1(Phi) -> Signal Specification/1
  "X_a(t)\t"/1 -> Bus Selector/1, Create M/1("X_a "), MATLAB Function/1(X_a)
  Create M/1(M) -> MATLAB Function/5(M)
  V/1 -> Selector/1, MATLAB Function/6(V)
  Signal Specification/1 -> Phi/1
  Bus Selector/1 -> Create Rotation Matrix 1/1(q)  "<ieps>"
  Create Rotation Matrix 1/1(R) -> Math Function/1
  Selector/1 -> Product/2
  Product/1 -> MATLAB Function/7(om_EE)
  Math Function/1 -> Product/1

== system EKF_SIL_02_newdelIpsOOSM/EKF/OOSM_KF/OOSM_enable/Create nominal q ==
  timestamp_meas : Inport
  Trigger : TriggerPort  PortDimensions=1
  Constant : Constant  Value=[0]
  Data Store Read : DataStoreRead  DialogController=Simulink.DDGSource  DataStoreName=lastUpdate_X_a  DataStoreElements=lastUpdate_X_a
  Data Store Read1 : DataStoreRead  DataStoreName=last_update_timestamp
  Delay1 : Delay  DelayLength=1  InitialConditionSource=Input port  InitialCondition=0
      settings: InputPortMap=u0,p4
  Digital Clock : DigitalClock  SampleTime=-1
  Display{,1..5} (6 alike) : Display
  Gain : Gain  Gain=0.5
  IC1 : InitialCondition  Value=X_a_0(1:4)
  MATLAB Function : MATLAB Function  TreatAsAtomicUnit=on
      settings: PermitHierarchicalResolution=ParametersOnly
  Matrix Exponential : dspmtrx3/Matrix Exponential
  Product : Product
  Product1 : Product  Multiplication=Matrix(*)
  Selector : Selector  InputPortWidth=20  Indices=[1:4]
  Selector1 : Selector  InputPortWidth=20  Indices=[5:7]
  Sum : Sum  Inputs=|+-
  Vector Concatenate : Concatenate
  flag : Constant  Value=0
  q(0) : Constant  Value=X_a_0(1:4)
  t_begin : Constant  Value=0
  "t_delta " : Constant  Value=t_delta
  q_nominal : Outport
  wires:
  MATLAB Function/1(CrossTensor) -> Product/1
  Sum/1 -> Display2/1, Product/2
  Selector1/1 -> Vector Concatenate/1
  Constant/1 -> Vector Concatenate/2
  flag/1 -> MATLAB Function/2(flag)
  Product/1 -> Gain/1
  Vector Concatenate/1 -> MATLAB Function/1(q)
  Product1/1 -> IC1/1
  Gain/1 -> Matrix Exponential/1
  Matrix Exponential/1 -> Product1/1
  IC1/1 -> Display/1, q_nominal/1
  Selector/1 -> Product1/2, Display1/1
  Data Store Read/1 -> Display4/1, Selector1/1, Selector/1
  Digital Clock/1 -> Display3/1, Delay1/1, Sum/1
  Data Store Read1/1 -> Display5/1, Sum/2
  t_begin/1 -> Delay1/2

== system EKF_SIL_02_newdelIpsOOSM/EKF/OOSM_KF/OOSM_enable/Create nominal q2 ==
  timestamp_meas : Inport
  omega_robot : Inport  Port=2
  Trigger : TriggerPort  PortDimensions=1
  Constant : Constant  Value=[0]
  Data Store Read : DataStoreRead  DialogController=Simulink.DDGSource  DataStoreName=lastUpdate_X_a  DataStoreElements=lastUpdate_X_a
  Data Store Read1 : DataStoreRead  DataStoreName=last_update_timestamp
  Delay1 : Delay  DelayLength=1  InitialConditionSource=Input port  InitialCondition=0
      settings: InputPortMap=u0,p4
  Delay2 : Delay  DelayLength=1  InitialConditionSource=Input port  InitialCondition=0
      settings: InputPortMap=u0,p4
  Display{1..5} (5 alike) : Display
  Gain : Gain  Gain=0.5
  IC1 : InitialCondition  Value=X_a_0(17:20)
  MATLAB Function : MATLAB Function  TreatAsAtomicUnit=on
      settings: PermitHierarchicalResolution=ParametersOnly
  Matrix Exponential : dspmtrx3/Matrix Exponential
  Product : Product
  Product1 : Product  Multiplication=Matrix(*)
  Scope : Scope
      settings: SaveName=ScopeData23
  Selector1 : Selector  InputPortWidth=20  Indices=[17:20]
  Sum : Sum  Inputs=|+-
  Vector Concatenate : Concatenate
  flag : Constant
  t_begin : Constant  Value=0
  t_begin1 : Constant  Value=[0;0;0]
  "t_delta " : Constant  Value=t_delta
  ieps_nominal : Outport
  wires:
  t_begin/1 -> Delay1/2
  Data Store Read1/1 -> Sum/2, Display5/1
  timestamp_meas/1 -> Sum/1, Delay1/1, Display3/1
  Selector1/1 -> Display1/1, Product1/2
  IC1/1 -> ieps_nominal/1
  Matrix Exponential/1 -> Product1/1
  Gain/1 -> Matrix Exponential/1
  Product1/1 -> IC1/1
  Vector Concatenate/1 -> MATLAB Function/1(q)
  Product/1 -> Gain/1
  flag/1 -> MATLAB Function/2(flag)
  Constant/1 -> Vector Concatenate/2
  Sum/1 -> Product/2, Display2/1
  MATLAB Function/1(CrossTensor) -> Product/1
  Data Store Read/1 -> Selector1/1
  t_begin1/1 -> Delay2/2
  Delay2/1 -> Vector Concatenate/1, Display4/1
  omega_robot/1 -> Delay2/1

== system EKF_SIL_02_newdelIpsOOSM/EKF/OOSM_KF/OOSM_enable/Enabled Subsystem ==
  Enable : EnablePort
  Create H_k : Subsystem
  Data Store Read : DataStoreRead  DataStoreName=q_nominal_d
  "rho " : Constant  Value=rho
  wires:
  "rho "/1 -> Create H_k/1(rho)
  Data Store Read/1 -> Create H_k/2(q_nominal)

== system EKF_SIL_02_newdelIpsOOSM/EKF/OOSM_KF/Subsystem/Dynamic Model (Differential equations)2 ==
  X_a(t) : Inport
  "V " : Inport  Port=2
  Dynamic Model (Differential equations) : Subsystem
  X_a_dot : Outport
  wires:
  X_a(t)/1 -> Dynamic Model (Differential equations)/1(X_a(t))
  Dynamic Model (Differential equations)/1(X_a(t+1)) -> X_a_dot/1
  "V "/1 -> Dynamic Model (Differential equations)/2("V ")

== system EKF_SIL_02_newdelIpsOOSM/EKF/Predictor/Create State error covariance (P)/Process noise covariance [rotational] ==
  Phi : Inport
  Process Noise covariance : MATLAB Function  TreatAsAtomicUnit=on
      settings: PermitHierarchicalResolution=ParametersOnly
  p : Constant  Value=[p_x;p_y;p_z]
  sig_tau : Constant  Value=sig_tau
  t_delta : Constant  Value=t_Kalman
  Q_r : Outport
  wires:
  Phi/1 -> Process Noise covariance/1(Phi)
  t_delta/1 -> Process Noise covariance/3(t_delta)
  sig_tau/1 -> Process Noise covariance/4(tau)
  p/1 -> Process Noise covariance/6(p)
  Process Noise covariance/1(Q_r) -> Q_r/1

== system EKF_SIL_02_newdelIpsOOSM/EKF/Predictor/Create State error covariance (P)/Process noise covariance [translational] ==
  Process noise covariance [translational] : MATLAB Function  TreatAsAtomicUnit=on
      settings: PermitHierarchicalResolution=ParametersOnly
  n : Constant  Value=n
  sig_f : Constant  Value=sig_f
  t_Kalman : Constant  Value=t_Kalman
  Q_t : Outport
  wires:
  n/1 -> Process noise covariance [translational]/2(n)
  t_Kalman/1 -> Process noise covariance [translational]/1(t_Kalman)
  sig_f/1 -> Process noise covariance [translational]/3(sigma_f)
  Process noise covariance [translational]/1(Q_t_k) -> Q_t/1

== system EKF_SIL_02_newdelIpsOOSM/EKF/Predictor/Create State error covariance (P)/State Propagation ==
  "X_a(t)\t" : Inport
  V : Inport  Port=2
  Bus Selector : BusSelector  OutputSignals=ieps
  Create M : Subsystem
  Create Rotation Matrix 1 : Subsystem
  MATLAB Function : MATLAB Function  TreatAsAtomicUnit=on
      settings: PermitHierarchicalResolution=ParametersOnly
  Math Function : Math  Operator=transpose  SaturateOnIntegerOverflow=on
  Product : Product  Multiplication=Matrix(*)
  Selector : Selector  InputPortWidth=6  Indices=[4:6]
  Signal Specification : SignalSpecification  Dimensions=[18,18]
  n : Constant  Value=n
  p : Constant  Value=[p_x;p_y;p_z]
  "t_Kalman " : Constant  Value=t_Kalman
  Phi : Outport
  wires:
  p/1 -> Create M/2(p), MATLAB Function/4(p)
  n/1 -> MATLAB Function/2(n)
  "t_Kalman "/1 -> MATLAB Function/3(t_Kalman)
  MATLAB Function/1(Phi) -> Signal Specification/1
  "X_a(t)\t"/1 -> Bus Selector/1, Create M/1("X_a "), MATLAB Function/1(X_a)
  Create M/1(M) -> MATLAB Function/5(M)
  V/1 -> Selector/1, MATLAB Function/6(V)
  Signal Specification/1 -> Phi/1
  Bus Selector/1 -> Create Rotation Matrix 1/1(q)  "<ieps>"
  Create Rotation Matrix 1/1(R) -> Math Function/1
  Selector/1 -> Product/2
  Product/1 -> MATLAB Function/7(om_EE)
  Math Function/1 -> Product/1

== system EKF_SIL_02_newdelIpsOOSM/EKF/Predictor/Integrator/Dynamic Model (Differential equations)2 ==
  X_a(t) : Inport
  "V " : Inport  Port=2
  Dynamic Model (Differential equations) : Subsystem
  X_a_dot : Outport
  wires:
  X_a(t)/1 -> Dynamic Model (Differential equations)/1(X_a(t))
  Dynamic Model (Differential equations)/1(X_a(t+1)) -> X_a_dot/1
  "V "/1 -> Dynamic Model (Differential equations)/2("V ")

== system EKF_SIL_02_newdelIpsOOSM/Plant/Dynamic Model (Differential equations)/Orbital Dynamics /Create Skew Symmetric ==
  vector : Inport
  0 : Constant  Value=0
  Create 3x3 matrix : Subsystem
  Demux : Demux  Outputs=3
  Demux1 : Demux  Outputs=3
  Gain : Gain  Gain=-1
  skew symmetric Matrix : Outport
  wires:
  0/1 -> Create 3x3 matrix/1(a11), Create 3x3 matrix/5(a22), Create 3x3 matrix/9(a33)
  Demux/3 -> Create 3x3 matrix/2(a12)
  Demux1/2 -> Create 3x3 matrix/3(a13)
  Demux1/3 -> Create 3x3 matrix/4(a21)
  Demux/1 -> Create 3x3 matrix/6(a23)
  vector/1 -> Demux1/1, Gain/1
  Create 3x3 matrix/1(Matrix) -> skew symmetric Matrix/1
  Gain/1 -> Demux/1
  Demux/2 -> Create 3x3 matrix/7(a31)
  Demux1/1 -> Create 3x3 matrix/8(a32)

== system EKF_SIL_02_newdelIpsOOSM/Plant/Dynamic Model (Differential equations)/Orbital Dynamics /norm  ==
  vector : Inport
  Dot Product : DotProduct  InputSameDT=on  OutDataTypeStr=Inherit: Inherit via internal rule
  Sqrt : Sqrt  SaturateOnIntegerOverflow=on
  "norm " : Outport
  wires:
  Dot Product/1 -> Sqrt/1
  vector/1 -> Dot Product/2, Dot Product/1
  Sqrt/1 -> "norm "/1

== system EKF_SIL_02_newdelIpsOOSM/Plant/Dynamic Model (Differential equations)/Rotational Dynamics/Create  J ==
  p : Inport
  0 : Constant  Value=0
  1 : Constant
  Create 3x3 matrix : Subsystem
  Fcn : Fcn  Expr=1-u(2)/1+u(1)
  Fcn1 : Fcn  Expr=1+u(3)/1-u(1)
  "J_k " : Outport
  wires:
  Fcn/1 -> Create 3x3 matrix/5(a22)
  p/1 -> Fcn1/1, Fcn/1
  0/1 -> Create 3x3 matrix/2(a12), Create 3x3 matrix/3(a13), Create 3x3 matrix/4(a21), Create 3x3 matrix/6(a23), Create 3x3 matrix/7(a31), Create 3x3 matrix/8(a32)
  Create 3x3 matrix/1(Matrix) -> "J_k "/1
  Fcn1/1 -> Create 3x3 matrix/9(a33)
  1/1 -> Create 3x3 matrix/1(a11)

== system EKF_SIL_02_newdelIpsOOSM/Plant/Dynamic Model (Differential equations)/Rotational Dynamics/Create Psi ==
  "omega " : Inport
  p : Inport  Port=2
  Create Psi : Concatenate  NumInputs=3
  Demux : Demux  Outputs=3
  Demux1 : Demux  Outputs=3
  Product{,1..5} (6 alike) : Product
  Psi : Outport
  wires:
  Demux1/3 -> Product1/2, Product3/2
  p/1 -> Demux/1
  Demux/3 -> Product4/1
  Product4/1 -> Create Psi/3
  Demux1/1 -> Product5/2, Product3/1
  Demux1/2 -> Product1/1, Product5/1
  Product2/1 -> Create Psi/2
  Demux/1 -> Product/1
  Create Psi/1 -> Psi/1
  Demux/2 -> Product2/1
  Product/1 -> Create Psi/1
  Product1/1 -> Product/2
  Product5/1 -> Product4/2
  Product3/1 -> Product2/2
  "omega "/1 -> Demux1/1

== system EKF_SIL_02_newdelIpsOOSM/Plots and display/Create Measurements [Pose]1/Create Measurements [Position]/Create Rotation Matrix  ==
  q : Inport
  Add : Sum
  Add5 : Sum  Inputs=+++
  Constant1 : Constant  Value=-1
  Create Skew Symmetric : Subsystem
  Gain : Gain  Gain=2
  Gain1 : Gain  Gain=2
  Gain2 : Gain  Gain=2
  I : Constant  Value=eye(3,3)
  Math Function : Math  Operator=square  SaturateOnIntegerOverflow=on
  Math Function1 : Math  Operator=transpose  SaturateOnIntegerOverflow=on
  Product1 : Product
  Product2 : Product
  Product3 : Product  Multiplication=Matrix(*)
  Selector2 : Selector  NumberOfDimensions=2  InputPortWidth=3  IndexOptions=Index vector (dialog),Index vector (dialog)  Indices=[1 2 3],1  OutputSizes=1,1
  Selector3 : Selector  NumberOfDimensions=2  InputPortWidth=3  IndexOptions=Index vector (dialog),Index vector (dialog)  Indices=[4],1  OutputSizes=1,1
  R : Outport
  wires:
  q/1 -> Selector2/1, Selector3/1
  Add5/1 -> R/1
  Product3/1 -> Gain2/1
  Math Function1/1 -> Product3/2
  Product1/1 -> Add5/3
  Gain1/1 -> Product2/1
  Create Skew Symmetric/1(skew symmetric Matrix) -> Gain1/1
  Product2/1 -> Add5/2
  Gain2/1 -> Add5/1
  Selector2/1 -> Create Skew Symmetric/1(vector), Product3/1, Math Function1/1
  I/1 -> Product1/2
  Add/1 -> Product1/1
  Selector3/1 -> Math Function/1, Product2/2
  Constant1/1 -> Add/2
  Math Function/1 -> Gain/1
  Gain/1 -> Add/1

== system EKF_SIL_02_newdelIpsOOSM/Plots and display/Create Measurements [Pose]2/Create Measurements [Position]/Create Rotation Matrix  ==
  q : Inport
  Add : Sum
  Add5 : Sum  Inputs=+++
  Constant1 : Constant  Value=-1
  Create Skew Symmetric : Subsystem
  Gain : Gain  Gain=2
  Gain1 : Gain  Gain=2
  Gain2 : Gain  Gain=2
  I : Constant  Value=eye(3,3)
  Math Function : Math  Operator=square  SaturateOnIntegerOverflow=on
  Math Function1 : Math  Operator=transpose  SaturateOnIntegerOverflow=on
  Product1 : Product
  Product2 : Product
  Product3 : Product  Multiplication=Matrix(*)
  Selector2 : Selector  NumberOfDimensions=2  InputPortWidth=3  IndexOptions=Index vector (dialog),Index vector (dialog)  Indices=[1 2 3],1  OutputSizes=1,1
  Selector3 : Selector  NumberOfDimensions=2  InputPortWidth=3  IndexOptions=Index vector (dialog),Index vector (dialog)  Indices=[4],1  OutputSizes=1,1
  R : Outport
  wires:
  Gain/1 -> Add/1
  Math Function/1 -> Gain/1
  Constant1/1 -> Add/2
  Selector3/1 -> Product2/2, Math Function/1
  Add/1 -> Product1/1
  I/1 -> Product1/2
  Selector2/1 -> Math Function1/1, Product3/1, Create Skew Symmetric/1(vector)
  Gain2/1 -> Add5/1
  Product2/1 -> Add5/2
  Create Skew Symmetric/1(skew symmetric Matrix) -> Gain1/1
  Gain1/1 -> Product2/1
  Product1/1 -> Add5/3
  Math Function1/1 -> Product3/2
  Product3/1 -> Gain2/1
  Add5/1 -> R/1
  q/1 -> Selector3/1, Selector2/1

== system EKF_SIL_02_newdelIpsOOSM/Plots and display/Create Measurements [Pose]2/Create Measurements [Position]/Create Rotation Matrix 1 ==
  q : Inport
  Add : Sum
  Add5 : Sum  Inputs=+++
  Constant1 : Constant  Value=-1
  Create Skew Symmetric : Subsystem
  Gain : Gain  Gain=2
  Gain1 : Gain  Gain=2
  Gain2 : Gain  Gain=2
  I : Constant  Value=eye(3,3)
  Math Function : Math  Operator=square  SaturateOnIntegerOverflow=on
  Math Function1 : Math  Operator=transpose  SaturateOnIntegerOverflow=on
  Product1 : Product
  Product2 : Product
  Product3 : Product  Multiplication=Matrix(*)
  Selector2 : Selector  NumberOfDimensions=2  InputPortWidth=3  IndexOptions=Index vector (dialog),Index vector (dialog)  Indices=[1 2 3],1  OutputSizes=1,1
  Selector3 : Selector  NumberOfDimensions=2  InputPortWidth=3  IndexOptions=Index vector (dialog),Index vector (dialog)  Indices=[4],1  OutputSizes=1,1
  R : Outport
  wires:
  Gain/1 -> Add/1
  Math Function/1 -> Gain/1
  Constant1/1 -> Add/2
  Selector3/1 -> Product2/2, Math Function/1
  Add/1 -> Product1/1
  I/1 -> Product1/2
  Selector2/1 -> Math Function1/1, Product3/1, Create Skew Symmetric/1(vector)
  Gain2/1 -> Add5/1
  Product2/1 -> Add5/2
  Create Skew Symmetric/1(skew symmetric Matrix) -> Gain1/1
  Gain1/1 -> Product2/1
  Product1/1 -> Add5/3
  Math Function1/1 -> Product3/2
  Product3/1 -> Gain2/1
  Add5/1 -> R/1
  q/1 -> Selector3/1, Selector2/1

== system EKF_SIL_02_newdelIpsOOSM/EKF/Control Signal/Create Rotation Matrix 2/Create Skew Symmetric/Create 3x3 matrix ==
  a11 : Inport
  a12 : Inport  Port=2
  a13 : Inport  Port=3
  a21 : Inport  Port=4
  a22 : Inport  Port=5
  a23 : Inport  Port=6
  a31 : Inport  Port=7
  a32 : Inport  Port=8
  a33 : Inport  Port=9
  Math Function : Math  Operator=transpose  SaturateOnIntegerOverflow=on
  Reshape (9) to [3x3] column-major : Reshape  OutputDimensionality=Customize  OutputDimensions=[3,3]
  Vector Concatenate : Concatenate  NumInputs=9
  Matrix : Outport
  wires:
  a33/1 -> Vector Concatenate/9
  a22/1 -> Vector Concatenate/5
  Vector Concatenate/1 -> Reshape (9) to [3x3] column-major/1
  a11/1 -> Vector Concatenate/1
  a12/1 -> Vector Concatenate/2
  a13/1 -> Vector Concatenate/3
  a23/1 -> Vector Concatenate/6
  a31/1 -> Vector Concatenate/7
  a32/1 -> Vector Concatenate/8
  a21/1 -> Vector Concatenate/4
  Reshape (9) to [3x3] column-major/1 -> Math Function/1
  Math Function/1 -> Matrix/1

== system EKF_SIL_02_newdelIpsOOSM/EKF/Create Measurements [Pose]2/Create Measurements [Position]/Create Rotation Matrix /Create Skew Symmetric ==
  vector : Inport
  0 : Constant  Value=0
  Create 3x3 matrix : Subsystem
  Demux : Demux  Outputs=3
  Demux1 : Demux  Outputs=3
  Gain : Gain  Gain=-1
  skew symmetric Matrix : Outport
  wires:
  0/1 -> Create 3x3 matrix/5(a22), Create 3x3 matrix/9(a33), Create 3x3 matrix/1(a11)
  Demux/3 -> Create 3x3 matrix/2(a12)
  Demux1/2 -> Create 3x3 matrix/3(a13)
  Demux1/3 -> Create 3x3 matrix/4(a21)
  Demux/1 -> Create 3x3 matrix/6(a23)
  vector/1 -> Demux1/1, Gain/1
  Create 3x3 matrix/1(Matrix) -> skew symmetric Matrix/1
  Gain/1 -> Demux/1
  Demux/2 -> Create 3x3 matrix/7(a31)
  Demux1/1 -> Create 3x3 matrix/8(a32)

== system EKF_SIL_02_newdelIpsOOSM/EKF/Create Measurements [Pose]2/Create Measurements [Position]/Create Rotation Matrix 1/Create Skew Symmetric ==
  vector : Inport
  0 : Constant  Value=0
  Create 3x3 matrix : Subsystem
  Demux : Demux  Outputs=3
  Demux1 : Demux  Outputs=3
  Gain : Gain  Gain=-1
  skew symmetric Matrix : Outport
  wires:
  0/1 -> Create 3x3 matrix/5(a22), Create 3x3 matrix/9(a33), Create 3x3 matrix/1(a11)
  Demux/3 -> Create 3x3 matrix/2(a12)
  Demux1/2 -> Create 3x3 matrix/3(a13)
  Demux1/3 -> Create 3x3 matrix/4(a21)
  Demux/1 -> Create 3x3 matrix/6(a23)
  vector/1 -> Demux1/1, Gain/1
  Create 3x3 matrix/1(Matrix) -> skew symmetric Matrix/1
  Gain/1 -> Demux/1
  Demux/2 -> Create 3x3 matrix/7(a31)
  Demux1/1 -> Create 3x3 matrix/8(a32)

== system EKF_SIL_02_newdelIpsOOSM/EKF/Measurement Update/Create X from X_a/Create del_q [body]/q_star ==
  q : Inport
  Demux : Demux
  Mux : Mux  Inputs=3
  Mux1 : Mux  Inputs=2
  Unary Minus : UnaryMinus
  q_star : Outport
  wires:
  Unary Minus/1 -> Mux1/1
  Demux/2 -> Mux/2
  Mux/1 -> Unary Minus/1
  Demux/4 -> Mux1/2
  Demux/3 -> Mux/3
  q/1 -> Demux/1
  Demux/1 -> Mux/1
  Mux1/1 -> q_star/1

== system EKF_SIL_02_newdelIpsOOSM/EKF/Measurement Update/Create X from X_a/Create del_q [inertial]/q_star ==
  q : Inport
  Demux : Demux
  Mux : Mux  Inputs=3
  Mux1 : Mux  Inputs=2
  Unary Minus : UnaryMinus
  q_star : Outport
  wires:
  Unary Minus/1 -> Mux1/1
  Demux/2 -> Mux/2
  Mux/1 -> Unary Minus/1
  Demux/4 -> Mux1/2
  Demux/3 -> Mux/3
  q/1 -> Demux/1
  Demux/1 -> Mux/1
  Mux1/1 -> q_star/1

== system EKF_SIL_02_newdelIpsOOSM/EKF/Measurement Update/Update with K(k) and predict current state/Create H_k/Create Bus [State Vector] ==
  X : Inport
  Bus Creator{1..5,7} (6 alike) : BusCreator  Inputs=3
  Bus Creator6 : BusCreator  Inputs=6
  Demux1 : Demux  Outputs=18
  X_bus : Outport
  wires:
  Demux1/4 -> Bus Creator3/1  "omega_x"
  Bus Creator2/1 -> Bus Creator6/1  "del_q"
  Demux1/8 -> Bus Creator4/2  "r_y"
  Demux1/6 -> Bus Creator3/3  "omega_z"
  Demux1/7 -> Bus Creator4/1  "r_x"
  Demux1/10 -> Bus Creator5/1  "r_x_dot"
  Bus Creator3/1 -> Bus Creator6/2  "omega"
  Demux1/3 -> Bus Creator2/3  "del_q_3"
  Demux1/1 -> Bus Creator2/1  "del_q_1"
  Demux1/11 -> Bus Creator5/2  "r_y_dot"
  Demux1/12 -> Bus Creator5/3  "r_z_dot"
  Demux1/2 -> Bus Creator2/2  "del_q_2"
  Demux1/5 -> Bus Creator3/2  "omega_y"
  Demux1/9 -> Bus Creator4/3  "r_z"
  Bus Creator4/1 -> Bus Creator6/3  "r"
  Bus Creator5/1 -> Bus Creator6/4  "r_dot"
  Bus Creator6/1 -> X_bus/1
  X/1 -> Demux1/1
  Demux1/13 -> Bus Creator1/1  "rho_c_x"
  Demux1/14 -> Bus Creator1/2  "rho_c_y"
  Demux1/15 -> Bus Creator1/3  "rho_c_z"
  Demux1/16 -> Bus Creator7/1  "del_ieps_1"
  Demux1/17 -> Bus Creator7/2
  Demux1/18 -> Bus Creator7/3  "del_ips_3"
  Bus Creator1/1 -> Bus Creator6/5  "rho_c"
  Bus Creator7/1 -> Bus Creator6/6  "del_ips"

== system EKF_SIL_02_newdelIpsOOSM/EKF/Measurement Update/Update with K(k) and predict current state/Create H_k/Create Rotation Matrix  ==
  q : Inport
  Add : Sum
  Add5 : Sum  Inputs=+++
  Constant1 : Constant  Value=-1
  Create Skew Symmetric : Subsystem
  Gain : Gain  Gain=2
  Gain1 : Gain  Gain=2
  Gain2 : Gain  Gain=2
  I : Constant  Value=eye(3,3)
  Math Function : Math  Operator=square  SaturateOnIntegerOverflow=on
  Math Function1 : Math  Operator=transpose  SaturateOnIntegerOverflow=on
  Product1 : Product
  Product2 : Product
  Product3 : Product  Multiplication=Matrix(*)
  Selector2 : Selector  NumberOfDimensions=2  InputPortWidth=3  IndexOptions=Index vector (dialog),Index vector (dialog)  Indices=[1 2 3],1  OutputSizes=1,1
  Selector3 : Selector  NumberOfDimensions=2  InputPortWidth=3  IndexOptions=Index vector (dialog),Index vector (dialog)  Indices=[4],1  OutputSizes=1,1
  R : Outport
  wires:
  Gain/1 -> Add/1
  Math Function/1 -> Gain/1
  Constant1/1 -> Add/2
  Selector3/1 -> Product2/2, Math Function/1
  Add/1 -> Product1/1
  I/1 -> Product1/2
  Selector2/1 -> Math Function1/1, Product3/1, Create Skew Symmetric/1(vector)
  Gain2/1 -> Add5/1
  Product2/1 -> Add5/2
  Create Skew Symmetric/1(skew symmetric Matrix) -> Gain1/1
  Gain1/1 -> Product2/1
  Product1/1 -> Add5/3
  Math Function1/1 -> Product3/2
  Product3/1 -> Gain2/1
  Add5/1 -> R/1
  q/1 -> Selector3/1, Selector2/1

== system EKF_SIL_02_newdelIpsOOSM/EKF/Measurement Update/Update with K(k) and predict current state/Create H_k/Create Rotation Matrix 1 ==
  q : Inport
  Add : Sum
  Add5 : Sum  Inputs=+++
  Constant1 : Constant  Value=-1
  Create Skew Symmetric : Subsystem
  Gain : Gain  Gain=2
  Gain1 : Gain  Gain=2
  Gain2 : Gain  Gain=2
  I : Constant  Value=eye(3,3)
  Math Function : Math  Operator=square  SaturateOnIntegerOverflow=on
  Math Function1 : Math  Operator=transpose  SaturateOnIntegerOverflow=on
  Product1 : Product
  Product2 : Product
  Product3 : Product  Multiplication=Matrix(*)
  Selector2 : Selector  NumberOfDimensions=2  InputPortWidth=3  IndexOptions=Index vector (dialog),Index vector (dialog)  Indices=[1 2 3],1  OutputSizes=1,1
  Selector3 : Selector  NumberOfDimensions=2  InputPortWidth=3  IndexOptions=Index vector (dialog),Index vector (dialog)  Indices=[4],1  OutputSizes=1,1
  R : Outport
  wires:
  q/1 -> Selector2/1, Selector3/1
  Add5/1 -> R/1
  Product3/1 -> Gain2/1
  Math Function1/1 -> Product3/2
  Product1/1 -> Add5/3
  Gain1/1 -> Product2/1
  Create Skew Symmetric/1(skew symmetric Matrix) -> Gain1/1
  Product2/1 -> Add5/2
  Gain2/1 -> Add5/1
  Selector2/1 -> Create Skew Symmetric/1(vector), Product3/1, Math Function1/1
  I/1 -> Product1/2
  Add/1 -> Product1/1
  Selector3/1 -> Math Function/1, Product2/2
  Constant1/1 -> Add/2
  Math Function/1 -> Gain/1
  Gain/1 -> Add/1
